simulink model "quarter_sus_win"  (R2025a)
settings: Solver=FixedStepAuto  StartTime=0.0  StopTime=20  FixedStep=0.001  RelTol=1e-3
model workspace (MAT data in the model file):
  Cs : Simulink.Parameter (value not decoded)
  Cy_f1 = 128915.5
  Cy_r1 = 85943.6
  G0 : Simulink.Parameter (value not decoded)
  IDA_ISD_PBC_bd : Simulink.Parameter (value not decoded)
  IDA_ISD_PBC_c1 : Simulink.Parameter (value not decoded)
  IDA_ISD_PBC_k1 : Simulink.Parameter (value not decoded)
  IDA_ISD_PBC_k2 : Simulink.Parameter (value not decoded)
  IDA_ISD_PBC_r1 : Simulink.Parameter (value not decoded)
  IDA_PBC_cd4 = 2000
  IDA_PBC_kd2 = 10000
  IDA_PBC_r1 = 1.5
  IDA_PBC_r2 = 0.44
  ISD_1_b : Simulink.Parameter (value not decoded)
  ISD_1_c : Simulink.Parameter (value not decoded)
  ISD_1_k1 : Simulink.Parameter (value not decoded)
  ISD_1_k2 : Simulink.Parameter (value not decoded)
  Izz1 = 1536.7
  Ks : Simulink.Parameter (value not decoded)
  Kt : Simulink.Parameter (value not decoded)
  Q : Simulink.Parameter (value not decoded)
  Q_F : Simulink.Parameter (value not decoded)
  Q_b_deflec : Simulink.Parameter (value not decoded)
  Q_dot : Simulink.Parameter (value not decoded)
  Q_dot_s : Simulink.Parameter (value not decoded)
  Q_dot_s_h : Simulink.Parameter (value not decoded)
  Q_dot_u : Simulink.Parameter (value not decoded)
  Q_flec : Simulink.Parameter (value not decoded)
  Q_flec_t : Simulink.Parameter (value not decoded)
  SHADD_alpha : Simulink.Parameter (value not decoded)
  a1 = 1.015
  a_max : Simulink.Parameter (value not decoded)
  a_min : Simulink.Parameter (value not decoded)
  adva_max : Simulink.Parameter (value not decoded)
  adva_min : Simulink.Parameter (value not decoded)
  as_max : Simulink.Parameter (value not decoded)
  b1 = 1.895
  b_deflec : Simulink.Parameter (value not decoded)
  bump_height : Simulink.Parameter (value not decoded)
  bump_lenth : Simulink.Parameter (value not decoded)
  bump_start : Simulink.Parameter (value not decoded)
  damper_param : Simulink.Parameter (value not decoded)
  deflec_max : Simulink.Parameter (value not decoded)
  done_range : Simulink.Parameter (value not decoded)
  f0 : Simulink.Parameter (value not decoded)
  h1 = 0.54
  imp_Cs : Simulink.Parameter (value not decoded)
  imp_Ks : Simulink.Parameter (value not decoded)
  imp_Ms : Simulink.Parameter (value not decoded)
  inerter_b : Simulink.Parameter (value not decoded)
  inerter_b_2 : Simulink.Parameter (value not decoded)
  inerter_c : Simulink.Parameter (value not decoded)
  inerter_k : Simulink.Parameter (value not decoded)
  inerter_k_2 : Simulink.Parameter (value not decoded)
  ms : Simulink.Parameter (value not decoded)
  mu : Simulink.Parameter (value not decoded)
  noise_seed : Simulink.Parameter (value not decoded)
  omega_1 : Simulink.Parameter (value not decoded)
  omega_2 : Simulink.Parameter (value not decoded)
  omega_3 : Simulink.Parameter (value not decoded)
  omega_4 : Simulink.Parameter (value not decoded)
  punish_Q : Simulink.Parameter (value not decoded)
  punish_R : Simulink.Parameter (value not decoded)
  reward_w_as : Simulink.Parameter (value not decoded)
  reward_w_au : Simulink.Parameter (value not decoded)
  reward_w_defv : Simulink.Parameter (value not decoded)
  road_seed : Simulink.Parameter (value not decoded)
  road_type : Simulink.Parameter (value not decoded)
  sigma_f1 = 0.1
  sigma_r1 = 0.1
  sine_amp : Simulink.Parameter (value not decoded)
  sine_freq : Simulink.Parameter (value not decoded)
  u : Simulink.Parameter (value not decoded)
  vs0 : Simulink.Parameter (value not decoded)
  vu0 : Simulink.Parameter (value not decoded)
  x_max : Simulink.Parameter (value not decoded)
  x_min : Simulink.Parameter (value not decoded)
  xs0 : Simulink.Parameter (value not decoded)
  xu0 : Simulink.Parameter (value not decoded)
symbols that are objects in the model workspace (value not decoded): a_max, a_min, b_deflec, bump_height, bump_lenth, bump_start, Cs, damper_param, f0, G0, IDA_ISD_PBC_bd, IDA_ISD_PBC_c1, IDA_ISD_PBC_k1, IDA_ISD_PBC_k2, IDA_ISD_PBC_r1, imp_Cs, imp_Ks, imp_Ms, Ks, Kt, ms, mu, omega_1, omega_2, omega_3, omega_4, Q_b_deflec, Q_dot_s, Q_dot_s_h, Q_dot_u, Q_F, Q_flec, Q_flec_t, road_type, SHADD_alpha, sine_amp, sine_freq, vs0, vu0, xs0, xu0
undefined symbols (not defined in the file or in its folder): ADD, Force, IDA, Imp, PBC, SH, Train, Validation
libraries: fl_lib x32, nesl_utility x27, sdl_lib x2, deeplib x1, simulink x1
(part 6 of 6)

== matlab function quarter_sus_win/QuarterSuspension /Subsystem1/Semi Active Air Suspension simscape/Damper/semi-active/MATLAB Function1 ==
  data: displacement input; F_d output; velocity input; I input; params input
function F_d = improvedHystereticModel(displacement, velocity, I, params)
    % 从params数组中提取模型参数
    c1 = params(1); c2 = params(2); c3 = params(3);
    k1 = params(4); k2 = params(5); k3 = params(6);
    alpha1 = params(7); alpha2 = params(8);
    % f01 = params(9); f02 = params(10); f03 = params(11); % 这些参数似乎在模型中未使用
    gamma1 = params(12); gamma2 = params(13); gamma3 = params(14);
    beta = params(15); delta = params(16);

    % 根据I计算c, k, alpha, 和 gamma
    c = c1 * I^2 + c2 * I + c3;
    k = k1 * I^2 + k2 * I + k3;
    alpha = alpha1 * I + alpha2;
    gamma = gamma1 * I^2 + gamma2 * I + gamma3;

    % 计算c^*和z
    c_star = gamma * (sign(velocity) + 1);
    z = tanh(beta * velocity + delta * sign(displacement));

    % 计算减震器力
    F_d = (c + c_star) * velocity + k * displacement + alpha * z;
end

== matlab function quarter_sus_win/QuarterSuspension /reward_cal/reward_cal/cal_reward ==
  data: state_deflec input; b_def input; reward output; Q_flec input
function reward = fun_reward(state_deflec,b_def,Q_flec)

if state_deflec^2 - b_def^2 > -0.0002
    r_dflec = 1000;
else
    r_dflec = 1/2*log(b_def^2/(b_def^2-state_deflec^2));%定义动行程的BLF函数
end
% Q_r = blkdiag(Q,Q_dot);
% state_r  = [state_deflec,acc];
% reward = state * Q * state'+acc * Q_dot * acc'; %简单二次型reward 考虑加速度与四个状态
% reward  = state_r * Q_r * state_r'; %简单二次型 考虑加速度和动行程
reward = r_dflec * Q_flec; % 二次型加BLF组合

== matlab function quarter_sus_win/QuarterSuspension /Subsystem1/Semi Active Air Suspension/Damper/Hysteretic/MATLAB Function1 ==
  data: displacement input; F_d output; velocity input; I input; params input
function F_d = improvedHystereticModel(displacement, velocity, I, params)
    % 从params数组中提取模型参数
    c1 = params(1); c2 = params(2); c3 = params(3);
    k1 = params(4); k2 = params(5); k3 = params(6);
    alpha1 = params(7); alpha2 = params(8);
    % f01 = params(9); f02 = params(10); f03 = params(11); % 这些参数似乎在模型中未使用
    gamma1 = params(12); gamma2 = params(13); gamma3 = params(14);
    beta = params(15); delta = params(16);

    % 根据I计算c, k, alpha, 和 gamma
    c = c1 * I^2 + c2 * I + c3;
    k = k1 * I^2 + k2 * I + k3;
    alpha = alpha1 * I + alpha2;
    gamma = gamma1 * I^2 + gamma2 * I + gamma3;

    % 计算c^*和z
    c_star = gamma * (sign(velocity) + 1);
    z = tanh(beta * velocity + delta * sign(displacement));

    % 计算减震器力
    F_d = (c + c_star) * velocity + k * displacement + alpha * z;
end

== matlab function quarter_sus_win/QuarterSuspension /Subsystem1/Semi Active Air Suspension/Damper/Random Current/MATLAB Function1 ==
  data: displacement input; F_d output; velocity input; I input; params input
function F_d = improvedHystereticModel(displacement, velocity, I, params)
    % 从params数组中提取模型参数
    c1 = params(1); c2 = params(2); c3 = params(3);
    k1 = params(4); k2 = params(5); k3 = params(6);
    alpha1 = params(7); alpha2 = params(8);
    % f01 = params(9); f02 = params(10); f03 = params(11); % 这些参数似乎在模型中未使用
    gamma1 = params(12); gamma2 = params(13); gamma3 = params(14);
    beta = params(15); delta = params(16);

    % 根据I计算c, k, alpha, 和 gamma
    c = c1 * I^2 + c2 * I + c3;
    k = k1 * I^2 + k2 * I + k3;
    alpha = alpha1 * I + alpha2;
    gamma = gamma1 * I^2 + gamma2 * I + gamma3;

    % 计算c^*和z
    c_star = gamma * (sign(velocity) + 1);
    z = tanh(beta * velocity + delta * sign(displacement));

    % 计算减震器力
    F_d = (c + c_star) * velocity + k * displacement + alpha * z;
end

== matlab function quarter_sus_win/QuarterSuspension /Subsystem1/Semi Active Air Suspension/Damper/semi-active/MATLAB Function1 ==
  data: displacement input; F_d output; velocity input; I input; params input
function F_d = improvedHystereticModel(displacement, velocity, I, params)
    % 从params数组中提取模型参数
    c1 = params(1); c2 = params(2); c3 = params(3);
    k1 = params(4); k2 = params(5); k3 = params(6);
    alpha1 = params(7); alpha2 = params(8);
    % f01 = params(9); f02 = params(10); f03 = params(11); % 这些参数似乎在模型中未使用
    gamma1 = params(12); gamma2 = params(13); gamma3 = params(14);
    beta = params(15); delta = params(16);

    % 根据I计算c, k, alpha, 和 gamma
    c = c1 * I^2 + c2 * I + c3;
    k = k1 * I^2 + k2 * I + k3;
    alpha = alpha1 * I + alpha2;
    gamma = gamma1 * I^2 + gamma2 * I + gamma3;

    % 计算c^*和z
    c_star = gamma * (sign(velocity) + 1);
    z = tanh(beta * velocity + delta * sign(displacement));

    % 计算减震器力
    F_d = (c + c_star) * velocity + k * displacement + alpha * z;
end

== matlab function quarter_sus_win/QuarterSuspension /Variant Subsystem/Vaildation-Force/obsprocess ==
  data: state input; obs output
function obs = fun_done(state)
    obs = zeros(3,1);
    obs_scaling = [1.5, 20, 0.03];
    obs(1) = state(3)/obs_scaling(1);
    obs(2) = state(5)/obs_scaling(2);
    obs(3) = state(6)/obs_scaling(3);
%     for t=7:1:27
%         x = state(1) + delta_t*ref_v*(t-6);
%         obs(t) = ref_A(1)*sin(2*pi/ref_T(1)*x + ref_fai(1)) + ref_A(2)*sin(2*pi/ref_T(2)*x + ref_fai(2)) + ref_A(3)*sin(2*pi/ref_T(3)*x + ref_fai(3));
%     end

end

== matlab function quarter_sus_win/QuarterSuspension /Variant Subsystem/Vaildation-Imp/obsprocess ==
  data: state input; obs output
function obs = fun_done(state)
    obs = zeros(3,1);
    obs_scaling = [1.5, 20, 0.03];
    obs(1) = state(3)/obs_scaling(1);
    obs(2) = state(5)/obs_scaling(2);
    obs(3) = state(6)/obs_scaling(3);
%     for t=7:1:27
%         x = state(1) + delta_t*ref_v*(t-6);
%         obs(t) = ref_A(1)*sin(2*pi/ref_T(1)*x + ref_fai(1)) + ref_A(2)*sin(2*pi/ref_T(2)*x + ref_fai(2)) + ref_A(3)*sin(2*pi/ref_T(3)*x + ref_fai(3));
%     end

end

== matlab function quarter_sus_win/QuarterSuspension /Variant Subsystem/Vaildation-Imp/actprocess ==
  data: act input; real_act output
function real_act = fun_act(act)

real_act= act;
end

== matlab function quarter_sus_win/QuarterSuspension /road_profile/gp/MATLAB Function ==
  data: X input; u output; gp_sample input; x input
function u = u_fn(X, gp_sample, x)
    u = interp1(X, gp_sample, x, 'linear', 'extrap');
end

== matlab function quarter_sus_win/QuarterSuspension /Variant Subsystem/Vaildation-3para-feedback/Subsystem/GOPS_Bridge/actprocess ==
  data: act input; real_act output
function real_act = fun_act(act)

real_act= act;
end

== matlab function quarter_sus_win/QuarterSuspension /Variant Subsystem/Vaildation-3para-feedback/obsprocess ==
  data: state input; obs output
function obs = fun_done(state)
    obs = zeros(3,1);
    obs_scaling = [1.5, 20, 0.03];
    obs(1) = state(3)/obs_scaling(1);
    obs(2) = state(5)/obs_scaling(2);
    obs(3) = state(6)/obs_scaling(3);
%     for t=7:1:27
%         x = state(1) + delta_t*ref_v*(t-6);
%         obs(t) = ref_A(1)*sin(2*pi/ref_T(1)*x + ref_fai(1)) + ref_A(2)*sin(2*pi/ref_T(2)*x + ref_fai(2)) + ref_A(3)*sin(2*pi/ref_T(3)*x + ref_fai(3));
%     end

end

== matlab function quarter_sus_win/QuarterSuspension /Variant Subsystem/IDA-PBC/Subsystem/我的控制/MATLAB Function ==
  data: cs input; ks input; ct input; r1 input; u output; r2 input; kd2 input; cd4 input; q1 input; q2 input; dq1 input; dq2 input
function u = calculateEquation(cs, ks,ct, r1, r2, kd2,cd4, q1,q2,dq1,dq2)
    % Calculate each term of the equation
    term1 = (ks - r2*kd2)*q1;
    term2 = (r1 - r2)*kd2*q2 + cs*dq1;
    % term4 = r2 * (r2 - r1)* cd4;
    term3 = (cd4/2 - cd4/r2 + (2*cd4)/(-r1 + r2)+cs)*dq1;
    
    term5 = (cd4/2 - (cd4*r1)/(2*r2)) * dq2;

    % Sum all terms to get u
    u = term1 + term2 + term3 - term5;
end

== matlab function quarter_sus_win/QuarterSuspension /Variant Subsystem/PDD/Subsystem1/MATLAB Function ==
  data: Kxsvs input; y output; cmax input; cmin input; vdef input; xdef input; Cs input
function y = PDD_switch(Kxsvs,cmax,cmin,vdef, xdef,Cs)
vdef2 = vdef^2;
    if (Kxsvs + ((cmax + Cs) * vdef2)) < 0
        y = 1;
    elseif (vdef == 0) && (xdef ~= 0) 
        y = 3;
    elseif (Kxsvs + ((cmin +Cs) *vdef2)) >= 0
        y = 2;
    else
        y = 4 ;
    end
end
